simulink model "pblm1b"  (R2020b)
settings: Solver=VariableStepAuto  StartTime=0.0  StopTime=10.0  RelTol=1e-3
libraries: cstblocks x4
settings Model: Creator=Jonas  LastModifiedBy=Jonas

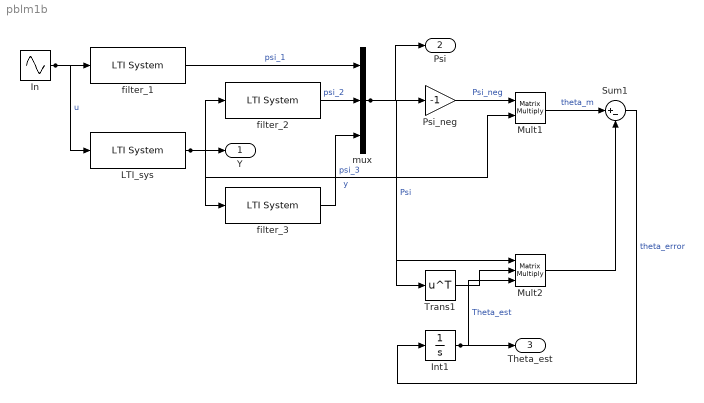
== system pblm1b ==
  In : Sin  SampleTime=0
  Int1 : Integrator
  LTI_sys : cstblocks/LTI System  sys=lti_sys  IC=x0
  Mult1 : Product  Inputs=**  Multiplication=Matrix(*)
  Mult2 : Product  Inputs=***  Multiplication=Matrix(*)
  Psi_neg : Gain  Gain=-1
  Sum1 : Sum  Inputs=|+-
  Trans1 : Math  Operator=transpose  SaturateOnIntegerOverflow=on
  filter_1 : cstblocks/LTI System  sys=filter_1  IC=[]
  filter_2 : cstblocks/LTI System  sys=filter_2  IC=[]
  filter_3 : cstblocks/LTI System  sys=filter_3  IC=[]
  mux : Mux  Inputs=3
  Y : Outport
  Psi : Outport  Port=2
  Theta_est : Outport  Port=3
  wires:
  Mult1/1 -> Sum1/1  "theta_m"
  Mult2/1 -> Sum1/2
  Int1/1 -> Mult2/3, Theta_est/1  "Theta_est"
  filter_2/1 -> mux/2  "psi_2"
  Trans1/1 -> Mult2/2
  filter_1/1 -> mux/1  "psi_1"
  filter_3/1 -> mux/3  "psi_3"
  Sum1/1 -> Int1/1  "theta_error"
  Psi_neg/1 -> Mult1/1  "Psi_neg"
  mux/1 -> Psi_neg/1, Trans1/1, Mult2/1, Psi/1  "Psi"
  LTI_sys/1 -> filter_2/1, filter_3/1, Mult1/2, Y/1  "y"
  In/1 -> LTI_sys/1, filter_1/1  "u"
